simulink model "proximity_sliding_mode_1"  (R2019b)
settings: Solver=VariableStepAuto  StartTime=0.0  StopTime=10  RelTol=1e-3
settings Model: Creator=Alien  LastModifiedBy=Alien
settings SolverCC: ZeroCrossAlgorithm=Adaptive  AlgebraicLoopSolver=LineSearch
settings DebuggingCC: IgnoredZcDiagnostic=none

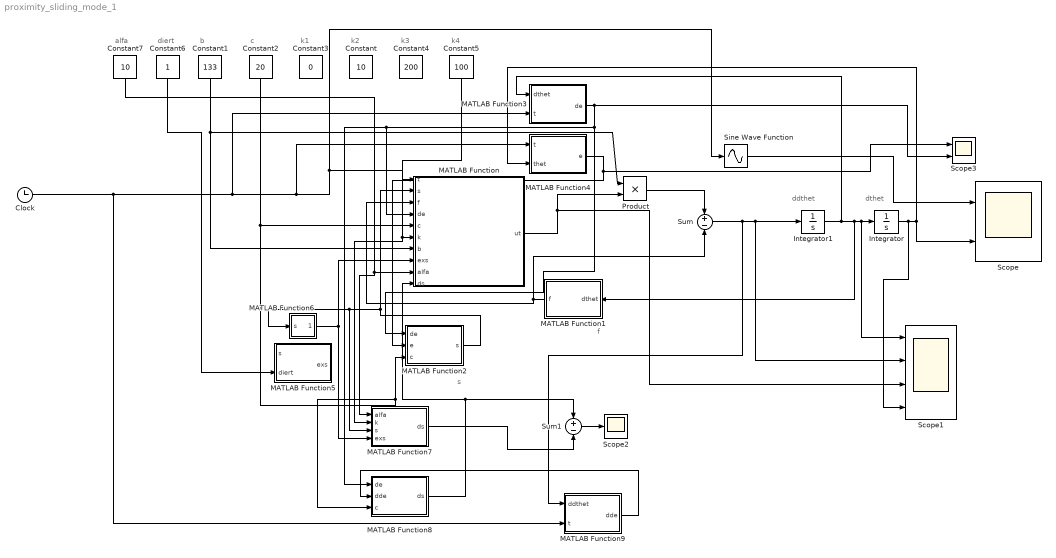
== system proximity_sliding_mode_1 ==
  note: diert
  note: s
  note: f
  note: k4
  note: k3
  note: k2
  note: k1
  note: c
  note: b
  note: dthet
  note: ddthet
  note: alfa
  Clock : Clock
  Constant : Constant  Value=10
  Constant1 : Constant  Value=133
  Constant2 : Constant  Value=20
  Constant3 : Constant  Value=0
  Constant4 : Constant  Value=200
  Constant5 : Constant  Value=100
  Constant6 : Constant
  Constant7 : Constant  Value=10
  Integrator : Integrator  InitialCondition=5
  Integrator1 : Integrator  InitialCondition=3
  MATLAB Function : MATLAB Function  TreatAsAtomicUnit=on
  MATLAB Function1 : MATLAB Function  TreatAsAtomicUnit=on
  MATLAB Function2 : MATLAB Function  TreatAsAtomicUnit=on
  MATLAB Function3 : MATLAB Function  TreatAsAtomicUnit=on
  MATLAB Function4 : MATLAB Function  TreatAsAtomicUnit=on
  MATLAB Function5 : MATLAB Function  TreatAsAtomicUnit=on
  MATLAB Function6 : MATLAB Function  TreatAsAtomicUnit=on
  MATLAB Function7 : MATLAB Function  TreatAsAtomicUnit=on
  MATLAB Function8 : MATLAB Function  TreatAsAtomicUnit=on
  MATLAB Function9 : MATLAB Function  TreatAsAtomicUnit=on
  Product : Product
  Scope : Scope  NumInputPorts=2
  Scope1 : Scope  NumInputPorts=4
  Scope2 : Scope
  Scope3 : Scope  NumInputPorts=2
  Sine Wave Function : Sin  TimeSource=Use external signal  SampleTime=0
  Sum : Sum  Inputs=+-
  Sum1 : Sum  Inputs=+-
  wires:
  Integrator1/1 -> MATLAB Function3/1(dthet), MATLAB Function1/1(dthet), Scope1/1, Integrator/1
  MATLAB Function1/1(f) -> Sum/2, MATLAB Function/3(f)
  Constant1/1 -> Product/1, MATLAB Function/7(b)
  Constant2/1 -> MATLAB Function2/3(c), MATLAB Function8/3(c), MATLAB Function/5(c)
  MATLAB Function4/1(e) -> Scope3/1, MATLAB Function2/2(e)
  MATLAB Function3/1(de) -> MATLAB Function8/1(de), MATLAB Function/4(de), MATLAB Function2/1(de), Scope3/2
  MATLAB Function/1(ut) -> Scope1/3, Product/2
  Integrator/1 -> Scope1/4, Scope/2, MATLAB Function4/2(thet)
  Product/1 -> Sum/1
  Sum/1 -> MATLAB Function9/1(ddthet), Scope1/2, Integrator1/1
  Clock/1 -> MATLAB Function9/2(t), MATLAB Function3/2(t), MATLAB Function4/1(t), Sine Wave Function/1, MATLAB Function/1(t)
  Sine Wave Function/1 -> Scope/1
  Constant5/1 -> MATLAB Function7/2(k), MATLAB Function/6(k)
  Constant6/1 -> MATLAB Function5/2(diert)
  Constant7/1 -> MATLAB Function7/1(alfa), MATLAB Function/9(alfa)
  MATLAB Function6/1(exs) -> MATLAB Function7/4(exs), MATLAB Function/8(exs)
  Sum1/1 -> Scope2/1
  MATLAB Function9/1(dde) -> MATLAB Function8/2(dde)
  MATLAB Function8/1(ds) -> MATLAB Function/10(ds), Sum1/1
  MATLAB Function2/1(s) -> MATLAB Function7/3(s), MATLAB Function6/1(s), MATLAB Function/2(s)
  MATLAB Function7/1(ds) -> Sum1/2

== matlab function proximity_sliding_mode_1/MATLAB Function1 ==
  data: dthet input; f output
function f = fcn(dthet)

f = 25 * dthet;

== matlab function proximity_sliding_mode_1/MATLAB Function ==
  data: t input; ut output; s input; f input; de input; c input; k input; b input; exs input; alfa input; ds input
function ut = fcn(t, s, f, de, c, k, b, exs, alfa, ds)
sigma = 5;

%dthet_d = cos(t);
ddthet_d = -sin(t);

ut = 1 / b * (de * c + ddthet_d + f + sigma * exs + k * s);
%ut = 1 / b * (de * c + ddthet_d + f + sigma * exs );
%ut = 1 / b * (de * c + ddthet_d + f + k * exs * (abs(s))^alfa);

end

== matlab function proximity_sliding_mode_1/MATLAB Function2 ==
  data: de input; s output; e input; c input
function s = fcn(de, e, c)
s = c*e + de;

== matlab function proximity_sliding_mode_1/MATLAB Function3 ==
  data: dthet input; de output; t input
function de = fcn(dthet, t)
%#codegen

de = cos(t) - dthet;

== matlab function proximity_sliding_mode_1/MATLAB Function4 ==
  data: t input; e output; thet input
function e = fcn(t, thet)

e = sin(t) - thet;

== matlab function proximity_sliding_mode_1/MATLAB Function5 ==
  data: s input; exs output; diert input
function exs = fcn(s, diert)
if s > diert
    exs = 1;
elseif s < diert
    exs = -1;
else
    exs = 1/diert*s;
end

== matlab function proximity_sliding_mode_1/MATLAB Function6 ==
  data: s input; exs output
function exs = fcn(s)
if s >= 0
    exs = 1;
else
    exs = -1;
end

== matlab function proximity_sliding_mode_1/MATLAB Function7 ==
  data: alfa input; ds output; k input; s input; exs input
function ds = fcn(alfa, k, s, exs)
sigma = 5;
ds = sigma * exs + k * s;
%ds = sigma * exs;
%ds = k * exs * (abs(s))^alfa;

== matlab function proximity_sliding_mode_1/MATLAB Function8 ==
  data: de input; ds output; dde input; c input
function ds = fcn(de, dde, c)
ds = c*de + dde;

== matlab function proximity_sliding_mode_1/MATLAB Function9 ==
  data: ddthet input; dde output; t input
function dde = fcn(ddthet, t)
%#codegen

dde = -sin(t) - ddthet;
